simulink model "Controle_aletas_novo"  (R2015a)
settings: Solver=ode45  StartTime=0.0  StopTime=10.0  RelTol=1e-3
values from neighbouring files (symbols this model uses):
  dt = 0.01    [untitled.m]
  I = Ki/Kp    (= 0.185294117647)    [RollControlParameters.m]
undefined symbols (not defined in the file or in its folder): Act2Aero, Aero2Act, b_ref, CD, Clalfa, Cldelta, Clp, Cmalfa, Cmq, Cnalfa, CXalfa, CYalfa, CZalfa, d_ref, dI, F, Kphi_1, Light, m, mass, MIL, qbar0, x_cg, x_ref
libraries: aerolibconvert2 x3, aerolibwind2 x3, aerolibasang x2, aerolibactuator x1, aerolib6dof2 x1, aerolibadyn x1, aerolibatmos2 x1
settings Model: Creator=Victor  LastModifiedBy=Victor

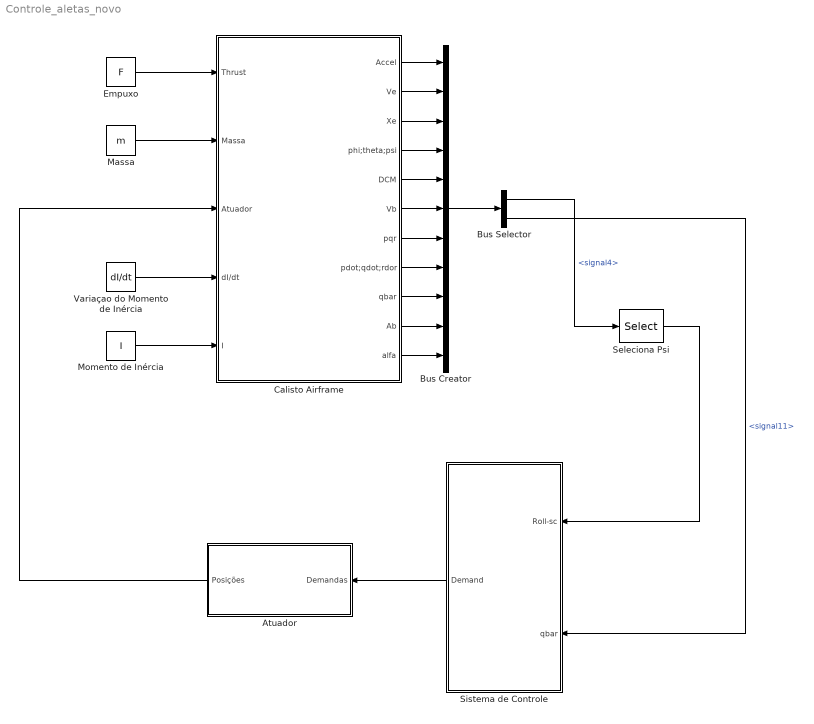
== system Controle_aletas_novo ==
  Atuador : Subsystem
  Bus Creator : BusCreator  Inputs=11
  Bus Selector : BusSelector  OutputSignals=signal4,signal11
  Calisto Airframe : Subsystem
  Empuxo : Constant  Value=F
  Massa : Constant  Value=m
  Momento de Inércia : Constant  Value=I
  Seleciona Psi : Selector  IndexMode=Zero-based  InputPortWidth=3  Indices=2
  Sistema de Controle : Subsystem
  Variaçao do Momento de Inércia : Constant  Value=dI/dt
  wires:
  Calisto Airframe/1(Accel) -> Bus Creator/1
  Calisto Airframe/2(Ve) -> Bus Creator/2
  Calisto Airframe/3(Xe) -> Bus Creator/3
  Calisto Airframe/4(phi;theta;psi) -> Bus Creator/4
  Calisto Airframe/5(DCM) -> Bus Creator/5
  Calisto Airframe/6(Vb) -> Bus Creator/6
  Calisto Airframe/7(pqr) -> Bus Creator/7
  Calisto Airframe/8(pdot;qdot;rdor) -> Bus Creator/8
  Calisto Airframe/9(qbar) -> Bus Creator/9
  Calisto Airframe/10(Ab) -> Bus Creator/10
  Calisto Airframe/11(alfa) -> Bus Creator/11
  Bus Creator/1 -> Bus Selector/1
  Bus Selector/2 -> Sistema de Controle/2(qbar)  "<signal11>"
  Sistema de Controle/1(Demand) -> Atuador/1(Demandas)
  Atuador/1(Posições) -> Calisto Airframe/3(Atuador)
  Variaçao do Momento de Inércia/1 -> Calisto Airframe/4(dI/dt)
  Momento de Inércia/1 -> Calisto Airframe/5(I)
  Massa/1 -> Calisto Airframe/2(Massa)
  Empuxo/1 -> Calisto Airframe/1(Thrust)
  Bus Selector/1 -> Seleciona Psi/1  "<signal4>"
  Seleciona Psi/1 -> Sistema de Controle/1(Roll-sc)

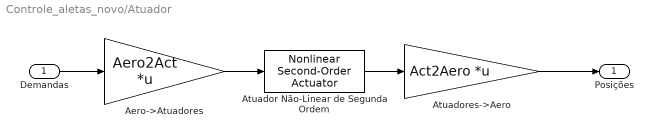
== system Controle_aletas_novo/Atuador ==
  Demandas : Inport
  Aero->Atuadores : Gain  Gain=Aero2Act  Multiplication=Matrix(K*u)  SaturateOnIntegerOverflow=on  OutDataTypeStr=Inherit: Same as input  ParamDataTypeStr=Inherit: Same as input
  Atuador Não-Linear de Segunda Ordem : aerolibactuator/Nonlinear Second-Order Actuator  wn_fin=wn_act  z_fin=z_act  fin_max=max_lim  fin_min=min_lim  fin_maxrate=inf  fin_act_0=0  fin_act_vel=0
  Atuadores->Aero : Gain  Gain=Act2Aero  Multiplication=Matrix(K*u)  SaturateOnIntegerOverflow=on  OutDataTypeStr=Inherit: Same as input  ParamDataTypeStr=Inherit: Same as input
  Posições : Outport
  wires:
  Demandas/1 -> Aero->Atuadores/1
  Aero->Atuadores/1 -> Atuador Não-Linear de Segunda Ordem/1
  Atuador Não-Linear de Segunda Ordem/1 -> Atuadores->Aero/1
  Atuadores->Aero/1 -> Posições/1

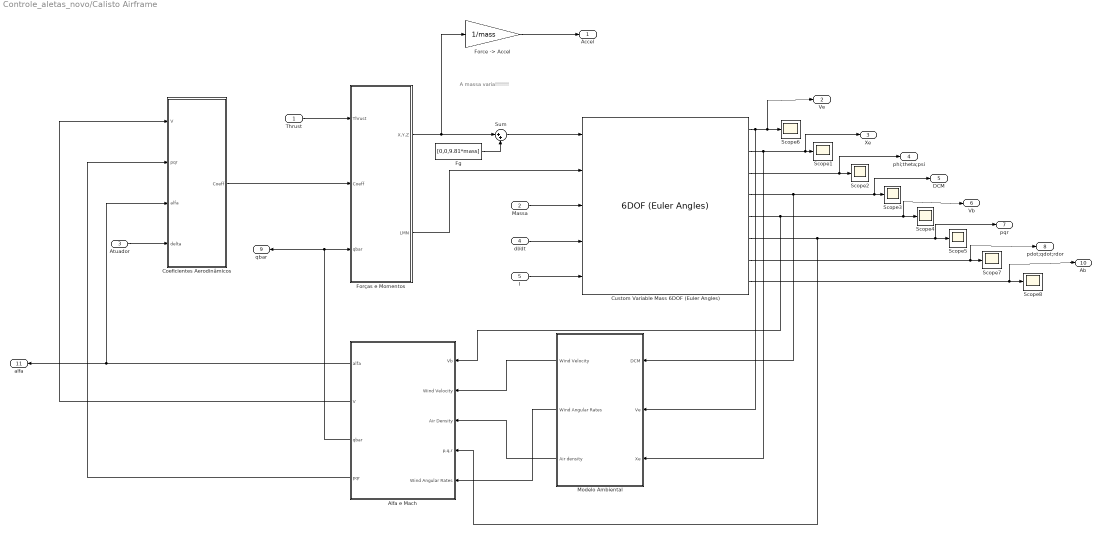
== system Controle_aletas_novo/Calisto Airframe ==
  note: A massa varia!!!!!!!
  Thrust : Inport
  Massa : Inport  Port=2
  Atuador : Inport  Port=3
  dI/dt : Inport  Port=4
  I : Inport  Port=5
  Alfa e Mach : Subsystem
  Coeficientes Aerodinâmicos : Subsystem
  Custom Variable Mass 6DOF (Euler Angles) : aerolib6dof2/6DOF (Euler Angles)  units=Metric (MKS)  mtype=Custom Variable  rep=Euler Angles  xme_0=[0 0 0]  Vm_0=[0 0 0]  eul_0=[0 0 0]  pm_0=[0 0 0]  mass_0=1.0  mass_e=0.5  mass_f=2.0  inertia=eye(3)  inertia_e=eye(3)  inertia_f=2*eye(3)  k_quat=1.0  vre_flag=off
  Fg : Constant  Value=[0,0,9.81*mass]
  "Force -> Accel" : Gain  Gain=1/mass
  Forças e Momentos : Subsystem
  Modelo Ambiental : Subsystem
  Scope{1..8} (8 alike) : Scope
      Scope2 settings: SaveName=ScopeData2
      Scope3 settings: SaveName=ScopeData3
      Scope4 settings: SaveName=ScopeData4
      Scope5 settings: SaveName=ScopeData5
      Scope7 settings: SaveName=ScopeData6
      Scope8 settings: SaveName=ScopeData7
  Sum : Sum  Inputs=|++  SaturateOnIntegerOverflow=on  InputSameDT=on  OutDataTypeStr=Inherit: Same as first input
  Accel : Outport
  Ve : Outport  Port=2
  Xe : Outport  Port=3
  phi;theta;psi : Outport  Port=4
  DCM : Outport  Port=5
  Vb : Outport  Port=6
  pqr : Outport  Port=7
  pdot;qdot;rdor : Outport  Port=8
  qbar : Outport  Port=9
  Ab : Outport  Port=10
  alfa : Outport  Port=11
  wires:
  Custom Variable Mass 6DOF (Euler Angles)/2 -> Modelo Ambiental/3(Xe), Scope1/1, Xe/1
  Custom Variable Mass 6DOF (Euler Angles)/4 -> Modelo Ambiental/1(DCM), Scope3/1, DCM/1
  Custom Variable Mass 6DOF (Euler Angles)/5 -> Alfa e Mach/1(Vb), Scope4/1, Vb/1
  Custom Variable Mass 6DOF (Euler Angles)/7 -> Scope7/1, pdot;qdot;rdor/1
  Custom Variable Mass 6DOF (Euler Angles)/8 -> Scope8/1, Ab/1
  Custom Variable Mass 6DOF (Euler Angles)/3 -> Scope2/1, phi;theta;psi/1
  Custom Variable Mass 6DOF (Euler Angles)/1 -> Modelo Ambiental/2(Ve), Scope6/1, Ve/1
  Custom Variable Mass 6DOF (Euler Angles)/6 -> Alfa e Mach/4(p,q,r), Scope5/1, pqr/1
  Forças e Momentos/2(LMN) -> Custom Variable Mass 6DOF (Euler Angles)/2
  Fg/1 -> Sum/2
  "Force -> Accel"/1 -> Accel/1
  Thrust/1 -> Forças e Momentos/1(Thrust)
  Coeficientes Aerodinâmicos/1(Coeff) -> Forças e Momentos/2(Coeff)
  Sum/1 -> Custom Variable Mass 6DOF (Euler Angles)/1
  Forças e Momentos/1(X,Y,Z) -> Sum/1, "Force -> Accel"/1
  Alfa e Mach/4(pqr) -> Coeficientes Aerodinâmicos/2(pqr)
  Atuador/1 -> Coeficientes Aerodinâmicos/4(delta)
  dI/dt/1 -> Custom Variable Mass 6DOF (Euler Angles)/4
  Massa/1 -> Custom Variable Mass 6DOF (Euler Angles)/3
  I/1 -> Custom Variable Mass 6DOF (Euler Angles)/5
  Modelo Ambiental/2(Wind Angular Rates) -> Alfa e Mach/5(Wind Angular Rates)
  Modelo Ambiental/1(Wind Velocity) -> Alfa e Mach/2(Wind Velocity)
  Modelo Ambiental/3(Air density) -> Alfa e Mach/3(Air Density)
  Alfa e Mach/3(qbar) -> qbar/1, Forças e Momentos/3(qbar)
  Alfa e Mach/2(V) -> Coeficientes Aerodinâmicos/1(V)
  Alfa e Mach/1(alfa) -> alfa/1, Coeficientes Aerodinâmicos/3(alfa)

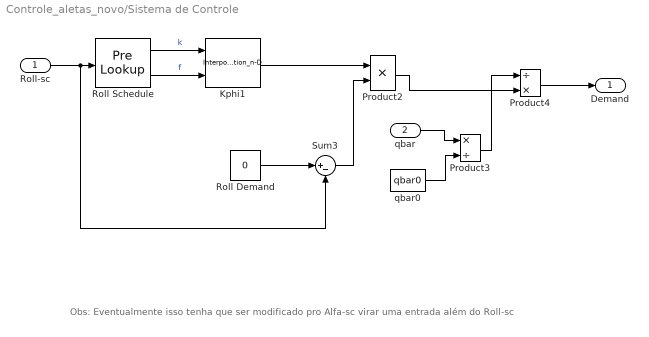
== system Controle_aletas_novo/Sistema de Controle ==
  note: Obs: Eventualmente isso tenha que ser modificado pro Alfa-sc virar uma entrada além do Roll-sc
  Roll-sc : Inport
  qbar : Inport  Port=2
  Kphi1 : Interpolation_n-D  NumberOfTableDimensions=1  Table=Kphi_1  RemoveProtectionIndex=on
      settings: InputPortMap=u0,u1
  Product2 : Product  SaturateOnIntegerOverflow=on  InputSameDT=on  OutDataTypeStr=Inherit: Same as first input
  Product3 : Product  Inputs=*/  SaturateOnIntegerOverflow=on  InputSameDT=on  OutDataTypeStr=Inherit: Same as first input
  Product4 : Product  Inputs=/*  SaturateOnIntegerOverflow=on  InputSameDT=on  OutDataTypeStr=Inherit: Same as first input
  Roll Schedule : PreLookup  BreakpointsData=a_vec  BeginIndexSearchUsingPreviousIndexResult=on  ExtrapMethod=Linear
  Roll Demand : Constant  Value=0
  Sum3 : Sum  Inputs=|+-  SaturateOnIntegerOverflow=on  InputSameDT=on  OutDataTypeStr=Inherit: Same as first input
  qbar0 : Constant  Value=qbar0
  Demand : Outport
  wires:
  Sum3/1 -> Product2/2
  Roll Demand/1 -> Sum3/1
  Roll-sc/1 -> Sum3/2, Roll Schedule/1
  Product4/1 -> Demand/1
  Roll Schedule/2 -> Kphi1/2  "f"
  Roll Schedule/1 -> Kphi1/1  "k"
  qbar0/1 -> Product3/2
  Product3/1 -> Product4/1
  qbar/1 -> Product3/1
  Product2/1 -> Product4/2
  Kphi1/1 -> Product2/1

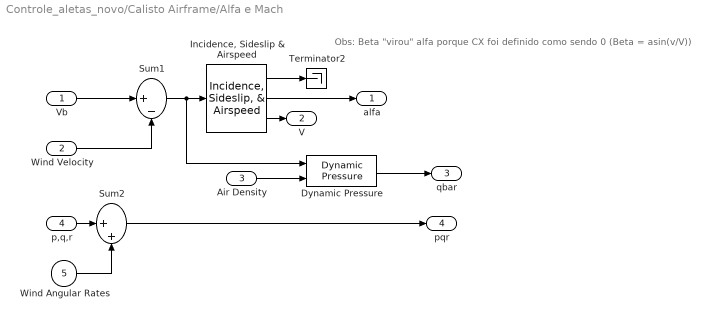
== system Controle_aletas_novo/Calisto Airframe/Alfa e Mach ==
  note: Obs: Beta "virou" alfa porque CX foi definido como sendo 0 (Beta = asin(v/V))
  Vb : Inport
  Wind Velocity : Inport  Port=2
  Air Density : Inport  Port=3
  p,q,r : Inport  Port=4
  Wind Angular Rates : Inport  Port=5
  Dynamic Pressure : aerolibasang/Dynamic Pressure
  "Incidence, Sideslip & Airspeed" : aerolibasang/Incidence, Sideslip, & Airspeed
  Sum1 : Sum  Inputs=|+-  SaturateOnIntegerOverflow=on  InputSameDT=on  OutDataTypeStr=Inherit: Same as first input
  Sum2 : Sum  Inputs=|++  SaturateOnIntegerOverflow=on  InputSameDT=on  OutDataTypeStr=Inherit: Same as first input
  Terminator2 : Terminator
  alfa : Outport
  V : Outport  Port=2
  qbar : Outport  Port=3
  pqr : Outport  Port=4
  wires:
  Wind Velocity/1 -> Sum1/2
  Vb/1 -> Sum1/1
  Air Density/1 -> Dynamic Pressure/2
  Dynamic Pressure/1 -> qbar/1
  "Incidence, Sideslip & Airspeed"/1 -> Terminator2/1
  "Incidence, Sideslip & Airspeed"/2 -> alfa/1
  "Incidence, Sideslip & Airspeed"/3 -> V/1
  Sum2/1 -> pqr/1
  p,q,r/1 -> Sum2/1
  Wind Angular Rates/1 -> Sum2/2
  Sum1/1 -> Dynamic Pressure/1, "Incidence, Sideslip & Airspeed"/1

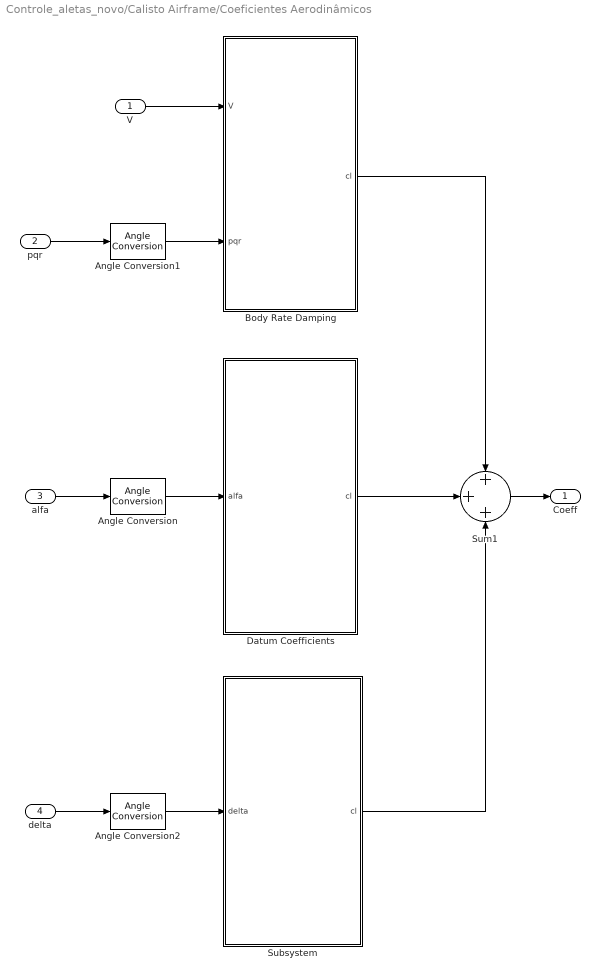
== system Controle_aletas_novo/Calisto Airframe/Coeficientes Aerodinâmicos ==
  V : Inport
  pqr : Inport  Port=2
  alfa : Inport  Port=3
  delta : Inport  Port=4
  Angle Conversion : aerolibconvert2/Angle Conversion  IU=rad  OU=deg
  Angle Conversion1 : aerolibconvert2/Angle Conversion  IU=rad  OU=deg
  Angle Conversion2 : aerolibconvert2/Angle Conversion  IU=rad  OU=deg
  Body Rate Damping : Subsystem
  Datum Coefficients : Subsystem
  Subsystem : Subsystem
  Sum1 : Sum  Inputs=+++  SaturateOnIntegerOverflow=on  InputSameDT=on  OutDataTypeStr=Inherit: Same as first input
  Coeff : Outport
  wires:
  pqr/1 -> Angle Conversion1/1
  V/1 -> Body Rate Damping/1(V)
  delta/1 -> Angle Conversion2/1
  Subsystem/1(cl) -> Sum1/3
  Sum1/1 -> Coeff/1
  alfa/1 -> Angle Conversion/1
  Body Rate Damping/1(cl) -> Sum1/1
  Datum Coefficients/1(cl) -> Sum1/2
  Angle Conversion/1 -> Datum Coefficients/1(alfa)
  Angle Conversion1/1 -> Body Rate Damping/2(pqr)
  Angle Conversion2/1 -> Subsystem/1(delta)

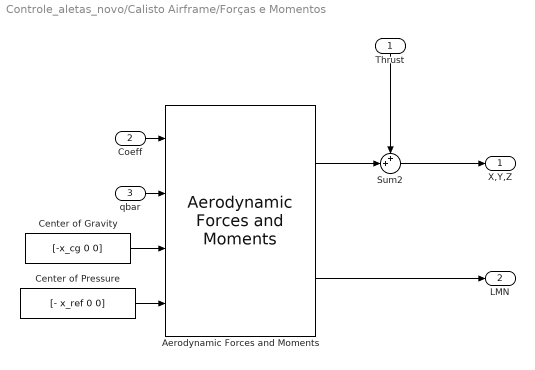
== system Controle_aletas_novo/Calisto Airframe/Forças e Momentos ==
  Thrust : Inport
  Coeff : Inport  Port=2
  qbar : Inport  Port=3
  Aerodynamic Forces and Moments : aerolibadyn/Aerodynamic Forces and Moments   inputAxes=Body  outputForceAxes=Body  outputMomentAxes=Body  S=1  b=1  cbar=1
  Center of Gravity : Constant  Value=[-x_cg 0 0]
  Center of Pressure : Constant  Value=[- x_ref 0 0]
  Sum2 : Sum  Inputs=++|  SaturateOnIntegerOverflow=on  InputSameDT=on  OutDataTypeStr=Inherit: Same as first input
  X,Y,Z : Outport
  LMN : Outport  Port=2
  wires:
  Coeff/1 -> Aerodynamic Forces and Moments/1
  Aerodynamic Forces and Moments/2 -> LMN/1
  qbar/1 -> Aerodynamic Forces and Moments/2
  Center of Gravity/1 -> Aerodynamic Forces and Moments/3
  Center of Pressure/1 -> Aerodynamic Forces and Moments/4
  Sum2/1 -> X,Y,Z/1
  Thrust/1 -> Sum2/1
  Aerodynamic Forces and Moments/1 -> Sum2/2

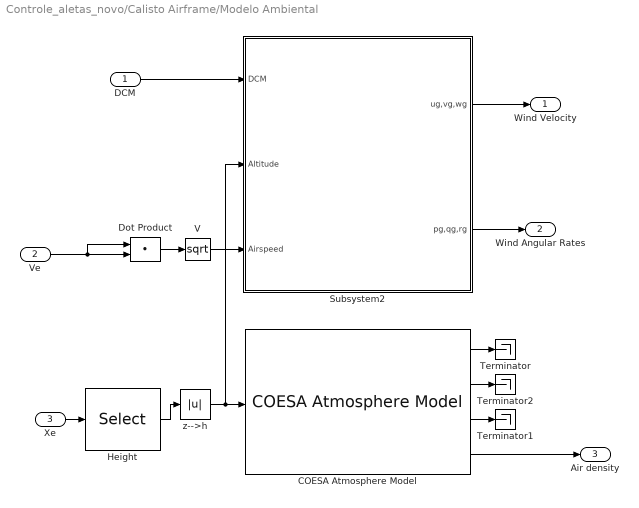
== system Controle_aletas_novo/Calisto Airframe/Modelo Ambiental ==
  DCM : Inport
  Ve : Inport  Port=2
  Xe : Inport  Port=3
  COESA Atmosphere Model : aerolibatmos2/COESA Atmosphere Model  units=Metric (MKS)  spec=1976 COESA-extended U.S. Standard Atmosphere  model=Profile  profile_var=High temperature  profile_percent=10%  profile_alt=5 km (16404 ft)  envelope_var=High temperature  envelope_percent=1%  action=None
  Dot Product : DotProduct  SaturateOnIntegerOverflow=on  OutDataTypeStr=Inherit: Inherit via internal rule
  Height : Selector  InputPortWidth=3  Indices=[3]
  Subsystem2 : Subsystem
  Terminator : Terminator
  Terminator1 : Terminator
  Terminator2 : Terminator
  V : Math  Operator=sqrt  SaturateOnIntegerOverflow=on
  z-->h : Abs  SaturateOnIntegerOverflow=on
  Wind Velocity : Outport
  Wind Angular Rates : Outport  Port=2
  Air density : Outport  Port=3
  wires:
  z-->h/1 -> Subsystem2/2(Altitude), COESA Atmosphere Model/1
  Subsystem2/1(ug,vg,wg) -> Wind Velocity/1
  Subsystem2/2(pg,qg,rg) -> Wind Angular Rates/1
  DCM/1 -> Subsystem2/1(DCM)
  Ve/1 -> Dot Product/1, Dot Product/2
  Dot Product/1 -> V/1
  V/1 -> Subsystem2/3(Airspeed)
  COESA Atmosphere Model/2 -> Terminator2/1
  COESA Atmosphere Model/3 -> Terminator1/1
  COESA Atmosphere Model/1 -> Terminator/1
  COESA Atmosphere Model/4 -> Air density/1
  Height/1 -> z-->h/1
  Xe/1 -> Height/1

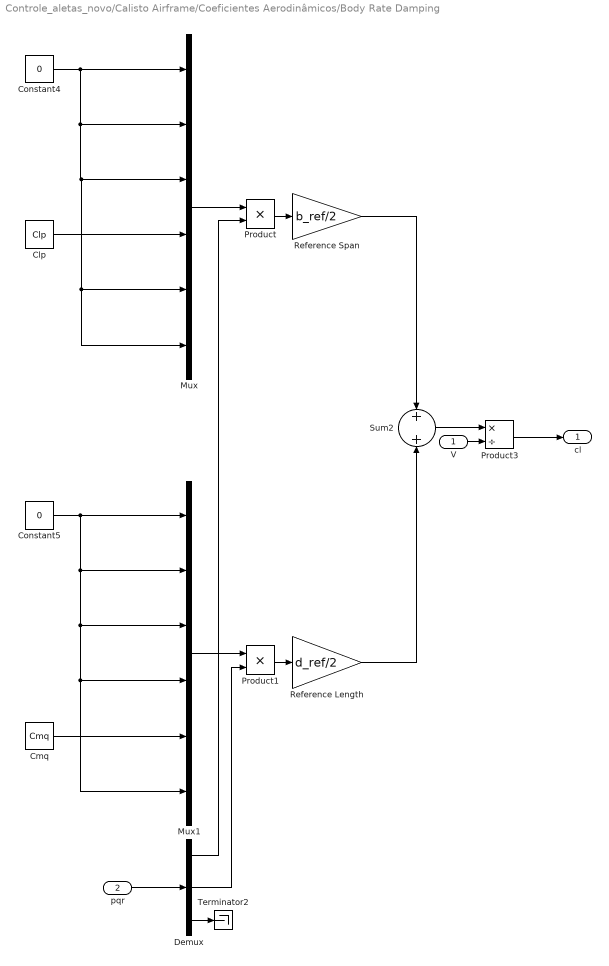
== system Controle_aletas_novo/Calisto Airframe/Coeficientes Aerodinâmicos/Body Rate Damping ==
  V : Inport
  pqr : Inport  Port=2
  Clp : Constant  Value=Clp
  Cmq : Constant  Value=Cmq
  Constant4 : Constant  Value=0
  Constant5 : Constant  Value=0
  Demux : Demux  Outputs=3
  Mux : Mux  Inputs=6
  Mux1 : Mux  Inputs=6
  Product : Product  SaturateOnIntegerOverflow=on  InputSameDT=on  OutDataTypeStr=Inherit: Same as first input
  Product1 : Product  SaturateOnIntegerOverflow=on  InputSameDT=on  OutDataTypeStr=Inherit: Same as first input
  Product3 : Product  Inputs=*/  SaturateOnIntegerOverflow=on  InputSameDT=on  OutDataTypeStr=Inherit: Same as first input
  Reference Length : Gain  Gain=d_ref/2  SaturateOnIntegerOverflow=on  OutDataTypeStr=Inherit: Same as input  ParamDataTypeStr=Inherit: Same as input
  Reference Span : Gain  Gain=b_ref/2  SaturateOnIntegerOverflow=on  OutDataTypeStr=Inherit: Same as input  ParamDataTypeStr=Inherit: Same as input
  Sum2 : Sum  SaturateOnIntegerOverflow=on  InputSameDT=on  OutDataTypeStr=Inherit: Same as first input
  Terminator2 : Terminator
  cl : Outport
  wires:
  Reference Length/1 -> Sum2/2
  Demux/3 -> Terminator2/1
  pqr/1 -> Demux/1
  Mux/1 -> Product/1
  Demux/2 -> Product1/2
  Demux/1 -> Product/2
  Constant5/1 -> Mux1/6, Mux1/4, Mux1/3, Mux1/2, Mux1/1
  Product1/1 -> Reference Length/1
  Mux1/1 -> Product1/1
  V/1 -> Product3/2
  Sum2/1 -> Product3/1
  Product3/1 -> cl/1
  Reference Span/1 -> Sum2/1
  Product/1 -> Reference Span/1
  Clp/1 -> Mux/4
  Constant4/1 -> Mux/6, Mux/5, Mux/3, Mux/2, Mux/1
  Cmq/1 -> Mux1/5

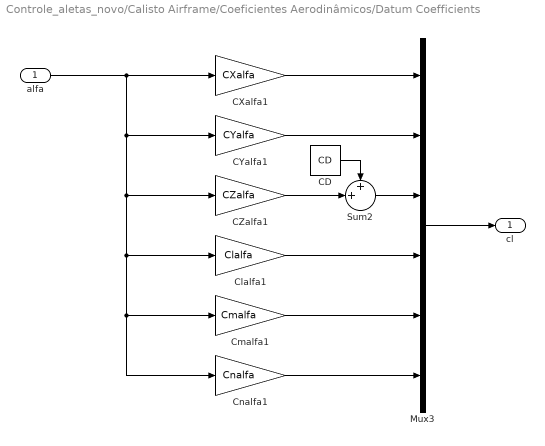
== system Controle_aletas_novo/Calisto Airframe/Coeficientes Aerodinâmicos/Datum Coefficients ==
  alfa : Inport
  CD : Constant  Value=CD
  CXalfa1 : Gain  Gain=CXalfa
  CYalfa1 : Gain  Gain=CYalfa
  CZalfa1 : Gain  Gain=CZalfa
  Clalfa1 : Gain  Gain=Clalfa
  Cmalfa1 : Gain  Gain=Cmalfa
  Cnalfa1 : Gain  Gain=Cnalfa
  Mux3 : Mux  Inputs=6
  Sum2 : Sum  Inputs=++|  SaturateOnIntegerOverflow=on  InputSameDT=on  OutDataTypeStr=Inherit: Same as first input
  cl : Outport
  wires:
  Mux3/1 -> cl/1
  Sum2/1 -> Mux3/3
  CD/1 -> Sum2/1
  CZalfa1/1 -> Sum2/2
  CYalfa1/1 -> Mux3/2
  Cmalfa1/1 -> Mux3/5
  Clalfa1/1 -> Mux3/4
  CXalfa1/1 -> Mux3/1
  alfa/1 -> Cnalfa1/1, Cmalfa1/1, Clalfa1/1, CZalfa1/1, CYalfa1/1, CXalfa1/1
  Cnalfa1/1 -> Mux3/6

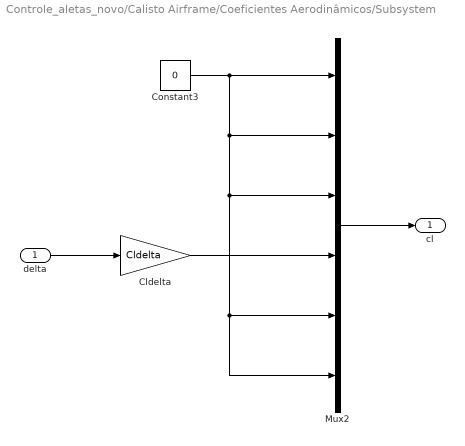
== system Controle_aletas_novo/Calisto Airframe/Coeficientes Aerodinâmicos/Subsystem ==
  delta : Inport
  Cldelta : Gain  Gain=Cldelta
  Constant3 : Constant  Value=0
  Mux2 : Mux  Inputs=6
  cl : Outport
  wires:
  Mux2/1 -> cl/1
  Cldelta/1 -> Mux2/4
  delta/1 -> Cldelta/1
  Constant3/1 -> Mux2/3, Mux2/5, Mux2/6, Mux2/2, Mux2/1

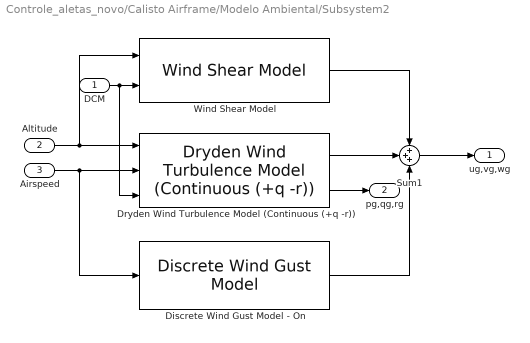
== system Controle_aletas_novo/Calisto Airframe/Modelo Ambiental/Subsystem2 ==
  DCM : Inport
  Altitude : Inport  Port=2
  Airspeed : Inport  Port=3
  Discrete Wind Gust Model - On : aerolibwind2/Discrete Wind Gust Model  units=Metric (MKS)  Gx=on  Gy=on  Gz=on  t_0=20  d_m=[120 120 80]  v_m=[3.5 3.0 3.0]
  Dryden Wind Turbulence Model (Continuous (+q -r)) : aerolibwind2/Dryden Wind Turbulence Model  (Continuous (+q -r))  units=Metric (MKS)  spec=MIL-F-8785C  model=Continuous Dryden (+q -r)  W20=5  Wdeg=0  TurbProb=10^-2 - Light  L_high=533.4  Wingspan=4  ts=0.1  Seed=[23341 23342 23343 23344]  T_on=on
  Sum1 : Sum  Inputs=+++  SaturateOnIntegerOverflow=on  InputSameDT=on  OutDataTypeStr=Inherit: Same as first input
  Wind Shear Model : aerolibwind2/Wind Shear Model  units=Metric (MKS)  phase=Category C - Terminal Flight Phase  W_20=1  Wdeg=0
  ug,vg,wg : Outport
  pg,qg,rg : Outport  Port=2
  wires:
  Dryden Wind Turbulence Model (Continuous (+q -r))/2 -> pg,qg,rg/1
  Wind Shear Model/1 -> Sum1/1
  Dryden Wind Turbulence Model (Continuous (+q -r))/1 -> Sum1/2
  Discrete Wind Gust Model - On/1 -> Sum1/3
  DCM/1 -> Dryden Wind Turbulence Model (Continuous (+q -r))/3, Wind Shear Model/2
  Airspeed/1 -> Dryden Wind Turbulence Model (Continuous (+q -r))/2, Discrete Wind Gust Model - On/1
  Sum1/1 -> ug,vg,wg/1
  Altitude/1 -> Dryden Wind Turbulence Model (Continuous (+q -r))/1, Wind Shear Model/1
